simulink model "AutomotiveEMS"  (R2018a)
settings: Solver=VariableStepAuto  StartTime=0  StopTime=3.5  FixedStep=1e-6
undefined symbols (not defined in the file): alternator, buck, DiscIntNeverNeededParam, electrical_load, hybrid_control, i_f_max, iceToAltRotRatio, n_ice_f, n_ice_i, rectifier, t_brake_f, t_brake_i, T_k, T_r, T_s
libraries: fl_lib x43, nesl_utility x41, elec_lib x33, simulink x10, SimscapeCustomBlocks_lib x2, dsparch4 x2, pe_lib x1
(part 2 of 3)

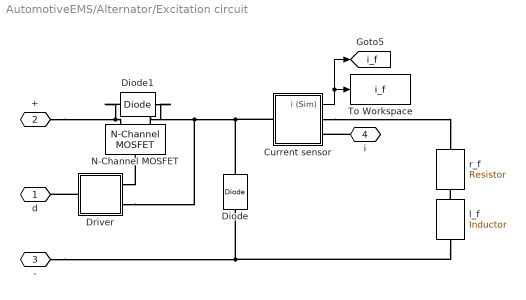
== system AutomotiveEMS/Alternator/Excitation circuit ==
  Current sensor : Subsystem
  Diode : elec_lib/Semiconductor Devices/Diode  ModelType=1  Vf=0.8 V  Ron=10e-3 Ohm  Goff=1e-8 S  Rz=0.3 Ohm  Vz=50 V  C_PWL=5 pF  prmExp=1  I12=[.0137, .545] A  V12=[.6, .7] V  I1=0.0137 A  V1=0.6 V  IS=1e-12 A  ec=1  RS=0.01 Ohm  Tmeas=25 degC  BV=inf V  C_param=1  CJ0=5 pF  VJ=1 V  Mgrad=0.5  Vvec=[.1, 10, 100] V  Cvec=[3.5, 1, .4] pF  FC=0.5  Q_param=1  Irrm=-7.15 A  iF=4 A  didt=-750 A/us  trr=115 ns  TT=50 ns  tau=100 ns  T_param=1  IS_T2=1.25e-7 A  I1_T2=0.245 A  V1_T2=0.5 V  Tmeas2=125 degC  EG_param=1  EG=1.11 eV  XTI_param=1  XTI=3  dBVdT=0 V/K  Tdevice=25 degC  i_capacitor_specify=off  i_capacitor_priority=High  i_capacitor=0 A  i_capacitor_nominal_specify=off  i_capacitor_nominal_unit=A  i_capacitor_nominal_value=1  v_capacitor_specify=off  v_capacitor_priority=None  v_capacitor=0 V  v_capacitor_nominal_specify=off  v_capacitor_nominal_unit=V  v_capacitor_nominal_value=1  Rth=[0, 10] K/W  thermal_mass_parameterization=1  thermal_mass=[0, 1] J/K  thermal_time_constant=[0, 10] s  thermal_mass_initial_temperatures=[25, 25] degC
      settings: SourceProductName=Simscape Electronics  SourceProductBaseCode=SN
  Diode1 : elec_lib/Semiconductor Devices/Diode  ModelType=1  Vf=0.8 V  Ron=10e-3 Ohm  Goff=1e-8 S  Rz=0.3 Ohm  Vz=50 V  C_PWL=5 pF  prmExp=1  I12=[.0137, .545] A  V12=[.6, .7] V  I1=0.0137 A  V1=0.6 V  IS=1e-12 A  ec=1  RS=0.01 Ohm  Tmeas=25 degC  BV=inf V  C_param=1  CJ0=5 pF  VJ=1 V  Mgrad=0.5  Vvec=[.1, 10, 100] V  Cvec=[3.5, 1, .4] pF  FC=0.5  Q_param=1  Irrm=-7.15 A  iF=4 A  didt=-750 A/us  trr=115 ns  TT=50 ns  tau=100 ns  T_param=1  IS_T2=1.25e-7 A  I1_T2=0.245 A  V1_T2=0.5 V  Tmeas2=125 degC  EG_param=1  EG=1.11 eV  XTI_param=1  XTI=3  dBVdT=0 V/K  Tdevice=25 degC  i_capacitor_specify=off  i_capacitor_priority=High  i_capacitor=0 A  i_capacitor_nominal_specify=off  i_capacitor_nominal_unit=A  i_capacitor_nominal_value=1  v_capacitor_specify=off  v_capacitor_priority=None  v_capacitor=0 V  v_capacitor_nominal_specify=off  v_capacitor_nominal_unit=V  v_capacitor_nominal_value=1  Rth=[0, 10] K/W  thermal_mass_parameterization=1  thermal_mass=[0, 1] J/K  thermal_time_constant=[0, 10] s  thermal_mass_initial_temperatures=[25, 25] degC
      settings: SourceProductName=Simscape Electronics  SourceProductBaseCode=SN
  Driver : Subsystem
  N-Channel MOSFET : elec_lib/Semiconductor Devices/N-Channel MOSFET  parameterization=1  prmDatasheet=1  prmEquCoeff=1  Beta=5 A/V^2  Rds=0.025 Ohm  Id=6 A  Vgs=alternator.rotor.s.v_gs_on V  Vth=1.7 V  lam=0 1/V  Tmeas=25 degC  RS=1e-4 Ohm  RD=0.01 Ohm  C_param=1  C_GS=270 pF  C_GD=80 pF  C_DS=0 pF  C_iss=350 pF  C_rss=80 pF  C_oss=0 pF  C_GS_vec=[ 270 300 290 280 295 255 ] pF  C_GD_vec=[ 450 400 300 190 95 55 ] pF  C_DS_vec=[ 450 410 390 230 175 115 ] pF  C_iss_vec=[ 720 700 590 470 390 310 ] pF  C_rss_vec=[ 450 400 300 190 95 55 ] pF  C_oss_vec=[ 900 810 690 420 270 170 ] pF  C_Vds_vec=[ 0.1 0.3 1 3 10 30 ] V  V_GS_for_cap_data=0 V  charge_linearity_param=1  C_OX=200 pF  V_C_OX=-0.5 V  IsDiode=0 A  Vbi=0.6 V  n=1  Cj0Diode=0 pF  TT=50e-9 s  dVth_dT=-6 mV/K  Rds_T2=0.037 Ohm  Tmeas2=125 degC  BEXDatasheet=-1.5  BEXEquCoeff=-1.5  etaisDatasheet=3  etaisEquCoeff=3  TdeviceDatasheet=25 degC  TdeviceEquCoeff=25 degC  Rth=[1, 10] K/W  thermal_mass_parameterization=1  thermal_mass=[1, 1] J/K  thermal_time_constant=[1, 10] s  thermal_mass_initial_temperatures=[ 25 25 ] degC  betaref=18 A/V^2  Vfbref=-1.1 V  gamma=3.5 V^0.50000  phib2ref=1 V  thesatref=0.4 1/V  alpha=0  Vp=5e-2 V  thesrref=0 1/V  m=8  Tref=25 degC  Cox=1500 pF  Cgso=100 pF  Cgdo=14 pF  Rsref=2e-3 Ohm  Rdref=0.17 Ohm  Rgref=8.4 Ohm  Isref=5.2e-13 A  Cj0=480 pF  Tprm=1  etabet=1.3  Stvfb=5e-4 V/K  Stphib=-8.5e-4 V/K  etasat=1.04  etasr=0.65  etar=0.95  etais=3  Tsim=25 degC  T0=[25, 25] degC
      settings: SourceProductName=Simscape Electronics  SourceProductBaseCode=SN
  To Workspace : ToWorkspace  VariableName=i_f  SaveFormat=Timeseries  SampleTime=-1
  l_f : elec_lib/Passive Devices/Inductor  l=alternator.rotor.l.value H  L_tol=20  enable_L_tol=0  tol_distribution=1  nSigma=4  r=0 Ohm  g=1e-9 1/Ohm  enable_operating_limits=0  operating_limit_action=2  max_working_current=1 A  power_rating=1 W  enable_faults=0  fault_action=1  lambdaPercent=50  k_faulted=0.9999  turnsShort=0  openCct=0  groundShort=0  groundShortG=0 1/Ohm  tau_fault=1e-3 s  enable_temporal_fault=0  t_fault=1 s  enable_behavioral_fault=0  max_permissible_voltage=100 V  n_fail_on_voltage=1  max_permissible_current=1 A  t_fail_on_current=1 s  i_L_specify=off  i_L_priority=High  i_L=0 A  i_L_nominal_specify=off  i_L_nominal_unit=A  i_L_nominal_value=1
      settings: SourceProductName=Simscape Electronics  SourceProductBaseCode=SN
  r_f : elec_lib/Passive Devices/Resistor  R=alternator.rotor.r.value Ohm  R_tol=5  enable_R_tol=0  tol_distribution=1  nSigma=4  enable_operating_limits=0  operating_limit_action=2  max_working_voltage=100 V  power_rating=1 W  enable_faults=0  fault_action=1  R_faulted=inf Ohm  enable_temporal_fault=0  t_fault=1 s  enable_behavioral_fault=0  max_permissible_current=1 A  t_fail_on_current=1 s  noise_mode=0  sample_time=1e-3 s  repeatability=1  auto_seed=2348512679  user_seed=0  Tdevice=25 degC  alpha=3.93e-3 1/K  Tmeas=25 degC  thermal_mass=100 J/K  power_derating_T1=70 degC  power_derating_T2=155 degC  operating_temperature_range_vec=[-50.0, 150.0] degC  temperature_specify=off  temperature_priority=High  temperature=298.15 K  temperature_nominal_specify=off  temperature_nominal_unit=K  temperature_nominal_value=1
  d : PMIOPort  Side=Left
  + : PMIOPort  Port=2  Side=Left
  - : PMIOPort  Port=3  Side=Left
  i : PMIOPort  Port=4  Side=Right
  tag scope: i_f=global
  wires:
  Current sensor/1(i (Sim)) -> [i_f], To Workspace/1
  connections:
  l_f/RConn1 -- Diode/LConn1 -- -/RConn1
  +/RConn1 -- Diode1/RConn1 -- N-Channel MOSFET/RConn1
  Current sensor/RConn1 -- r_f/RConn1
  Current sensor/LConn1 -- Diode/RConn1 -- Driver/RConn2 -- Diode1/LConn1 -- N-Channel MOSFET/RConn2
  l_f/LConn1 -- r_f/LConn1
  Driver/RConn1 -- N-Channel MOSFET/LConn1
  i/RConn1 -- Current sensor/RConn2
  Driver/LConn1 -- d/RConn1

== system AutomotiveEMS/Hybrid Load Matching Controller Scheme/Excitation current controller ==
  e : Inport
  on : Inport  Port=2
  Constant : Constant
  Fcn : Fcn  Expr=u > 0
  Switch : Switch  Criteria=u2 > Threshold  Threshold=0.5
  u : Outport
  wires:
  Switch/1 -> u/1
  on/1 -> Switch/2
  Constant/1 -> Switch/3
  Fcn/1 -> Switch/1
  e/1 -> Fcn/1

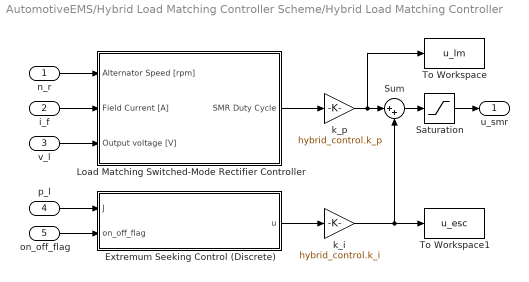
== system AutomotiveEMS/Hybrid Load Matching Controller Scheme/Hybrid Load Matching Controller ==
  n_r : Inport
  i_f : Inport  Port=2
  v_l : Inport  Port=3
  p_l : Inport  Port=4
  on_off_flag : Inport  Port=5
  Extremum Seeking Control (Discrete) : Subsystem  mask{a=0.025, f=sqrt(100*200), phi=180 - 4.2e-3/(1/sqrt(100*200))*360, K=0.25}
      mask prompts: a "Sine wave gain"; f "Sine wave frequency [Hz]"; phi "Sine wave phase [deg]"; K "Integrator gain"
      mask DialogControl ModParam Prompt: Modulation
      mask DialogControl IntegratorParam Prompt: Integrator
  Load Matching Switched-Mode Rectifier Controller : Subsystem  VariantControl=Variant  mask{p=alternator.p, u_lim_l=0.0, u_lim_u=1}
      mask prompts: p "Pole-pairs"; u_lim_l "Control signal lower limit"; u_lim_u "Control signal upper limit"
  Saturation : Saturate  UpperLimit=0.9  LowerLimit=0
  Sum : Sum  Inputs=|++
  To Workspace : ToWorkspace  VariableName=u_lm  SaveFormat=Timeseries  SampleTime=-1
  To Workspace1 : ToWorkspace  VariableName=u_esc  SaveFormat=Timeseries  SampleTime=-1
  k_i : Gain  Gain=hybrid_control.k_i
  k_p : Gain  Gain=hybrid_control.k_p
  u_smr : Outport
  wires:
  Extremum Seeking Control (Discrete)/1(u) -> k_i/1
  on_off_flag/1 -> Extremum Seeking Control (Discrete)/2(on_off_flag)
  i_f/1 -> Load Matching Switched-Mode Rectifier Controller/2(Field Current [A])
  Sum/1 -> Saturation/1
  Load Matching Switched-Mode Rectifier Controller/1(SMR Duty Cycle) -> k_p/1
  p_l/1 -> Extremum Seeking Control (Discrete)/1(J)
  v_l/1 -> Load Matching Switched-Mode Rectifier Controller/3(Output voltage [V])
  n_r/1 -> Load Matching Switched-Mode Rectifier Controller/1(Alternator Speed [rpm])
  Saturation/1 -> u_smr/1
  k_p/1 -> To Workspace/1, Sum/1
  k_i/1 -> To Workspace1/1, Sum/2

== system AutomotiveEMS/Mechanical speed/ICE Speed ==
  Ramp off : simulink/Sources/Ramp  slope=(s_f - s_i)/(t_f - t_i)  start=t_f  InitialOutput=0
  Ramp on : simulink/Sources/Ramp  slope=(s_f - s_i)/(t_f - t_i)  start=t_i  InitialOutput=s_i
  Sum : Sum  Inputs=+-
  s : Outport
  wires:
  Sum/1 -> s/1
  Ramp off/1 -> Sum/2
  Ramp on/1 -> Sum/1

== system AutomotiveEMS/Three-phase switched rectifier/Driver (S1) ==
  Controlled PWM Voltage : elec_lib/Actuators & Drivers/Drivers/Controlled PWM Voltage  F=rectifier.control.pwm.f_s Hz  TD=0 s  pulse_width_offset=0 s  pulse_min=0 s  Vmin=0 V  Vmax=5 V  Vm=5 V  pwm_or_av=1  event_type=2  sample_time=T_s s  u_min=0  u_max=1
      settings: SourceProductName=Simscape Electronics  SourceProductBaseCode=SN
  Electrical Reference : fl_lib/Electrical/Electrical Elements/Electrical Reference
  Gate Driver : elec_lib/Actuators & Drivers/Drivers/Gate Driver  vHigh=rectifier.s.v_gs_on*1.5 V  vLow=0 V  parameterization=1  rHigh=100 Ohm  rLow=10 Ohm  tRise=20 ns  tFall=20 ns  cLoad=10 nF  enable_faults=0  t_fault=1 s  fault_type=1  uHighValue=0.7  uLowValue=0.3  tHigh=50 ns  tLow=100 ns  ZonTime_specify=off  ZonTime_priority=None  ZonTime=0 s  ZoffTime_specify=off  ZoffTime_priority=None  ZoffTime=0 s  uHigh=2.0 V  uLow=0.8 V
      settings: SourceProductName=Simscape Electronics  SourceProductBaseCode=SN
  d : PMIOPort  Side=Left
  v_g : PMIOPort  Port=2  Side=Right
  v_s : PMIOPort  Port=3  Side=Right
  connections:
  Gate Driver/LConn2 -- Controlled PWM Voltage/RConn2 -- Electrical Reference/LConn1
  Controlled PWM Voltage/RConn1 -- Gate Driver/LConn1
  v_g/RConn1 -- Gate Driver/RConn1
  v_s/RConn1 -- Gate Driver/RConn2
  d/RConn1 -- Controlled PWM Voltage/LConn1

== system AutomotiveEMS/Three-phase switched rectifier/Driver (S2) ==
  Controlled PWM Voltage : elec_lib/Actuators & Drivers/Drivers/Controlled PWM Voltage  F=rectifier.control.pwm.f_s Hz  TD=0 s  pulse_width_offset=0 s  pulse_min=0 s  Vmin=0 V  Vmax=5 V  Vm=5 V  pwm_or_av=1  event_type=2  sample_time=T_s s  u_min=0  u_max=1
      settings: SourceProductName=Simscape Electronics  SourceProductBaseCode=SN
  Electrical Reference : fl_lib/Electrical/Electrical Elements/Electrical Reference
  Gate Driver : elec_lib/Actuators & Drivers/Drivers/Gate Driver  vHigh=rectifier.s.v_gs_on*1.5 V  vLow=0 V  parameterization=1  rHigh=100 Ohm  rLow=10 Ohm  tRise=20 ns  tFall=20 ns  cLoad=10 nF  enable_faults=0  t_fault=1 s  fault_type=1  uHighValue=0.7  uLowValue=0.3  tHigh=50 ns  tLow=100 ns  ZonTime_specify=off  ZonTime_priority=None  ZonTime=0 s  ZoffTime_specify=off  ZoffTime_priority=None  ZoffTime=0 s  uHigh=2.0 V  uLow=0.8 V
      settings: SourceProductName=Simscape Electronics  SourceProductBaseCode=SN
  d : PMIOPort  Side=Left
  v_g : PMIOPort  Port=2  Side=Right
  v_s : PMIOPort  Port=3  Side=Right
  connections:
  Gate Driver/LConn2 -- Controlled PWM Voltage/RConn2 -- Electrical Reference/LConn1
  Controlled PWM Voltage/RConn1 -- Gate Driver/LConn1
  v_g/RConn1 -- Gate Driver/RConn1
  v_s/RConn1 -- Gate Driver/RConn2
  d/RConn1 -- Controlled PWM Voltage/LConn1

== system AutomotiveEMS/Three-phase switched rectifier/Driver (S3) ==
  Controlled PWM Voltage : elec_lib/Actuators & Drivers/Drivers/Controlled PWM Voltage  F=rectifier.control.pwm.f_s Hz  TD=0 s  pulse_width_offset=0 s  pulse_min=0 s  Vmin=0 V  Vmax=5 V  Vm=5 V  pwm_or_av=1  event_type=2  sample_time=T_s s  u_min=0  u_max=1
      settings: SourceProductName=Simscape Electronics  SourceProductBaseCode=SN
  Electrical Reference : fl_lib/Electrical/Electrical Elements/Electrical Reference
  Gate Driver : elec_lib/Actuators & Drivers/Drivers/Gate Driver  vHigh=rectifier.s.v_gs_on*1.5 V  vLow=0 V  parameterization=1  rHigh=100 Ohm  rLow=10 Ohm  tRise=20 ns  tFall=20 ns  cLoad=10 nF  enable_faults=0  t_fault=1 s  fault_type=1  uHighValue=0.7  uLowValue=0.3  tHigh=50 ns  tLow=100 ns  ZonTime_specify=off  ZonTime_priority=None  ZonTime=0 s  ZoffTime_specify=off  ZoffTime_priority=None  ZoffTime=0 s  uHigh=2.0 V  uLow=0.8 V
      settings: SourceProductName=Simscape Electronics  SourceProductBaseCode=SN
  d : PMIOPort  Side=Left
  v_g : PMIOPort  Port=2  Side=Right
  v_s : PMIOPort  Port=3  Side=Right
  connections:
  Gate Driver/LConn2 -- Controlled PWM Voltage/RConn2 -- Electrical Reference/LConn1
  Controlled PWM Voltage/RConn1 -- Gate Driver/LConn1
  v_g/RConn1 -- Gate Driver/RConn1
  v_s/RConn1 -- Gate Driver/RConn2
  d/RConn1 -- Controlled PWM Voltage/LConn1

== system AutomotiveEMS/i_bus sensor/Current Sensor ==
  Ideal current sensor : Subsystem
  Noise addition : Subsystem  mask{T_s=T_s, seed=seed, noise=noise}
      mask prompts: T_s "Sample time [s]"; noise "Noise percentage"
  + : PMIOPort  Side=Left
  - : PMIOPort  Port=2  Side=Right
  m* : Outport
  m : Outport  Port=2
  wires:
  Ideal current sensor/1(i) -> m*/1, Noise addition/1(u)
  Noise addition/1(u + n) -> m/1
  connections:
  Ideal current sensor/RConn1 -- -/RConn1
  Ideal current sensor/LConn1 -- +/RConn1

== system AutomotiveEMS/i_l sensor/Current Sensor ==
  Ideal current sensor : Subsystem
  Noise addition : Subsystem  mask{T_s=T_s, seed=seed, noise=noise}
      mask prompts: T_s "Sample time [s]"; noise "Noise percentage"
  + : PMIOPort  Side=Left
  - : PMIOPort  Port=2  Side=Right
  m* : Outport
  m : Outport  Port=2
  wires:
  Ideal current sensor/1(i) -> m*/1, Noise addition/1(u)
  Noise addition/1(u + n) -> m/1
  connections:
  Ideal current sensor/RConn1 -- -/RConn1
  Ideal current sensor/LConn1 -- +/RConn1

== system AutomotiveEMS/i_uc sensor/Current Sensor ==
  Ideal current sensor : Subsystem
  Noise addition : Subsystem  mask{T_s=T_s, seed=seed, noise=noise}
      mask prompts: T_s "Sample time [s]"; noise "Noise percentage"
  + : PMIOPort  Side=Left
  - : PMIOPort  Port=2  Side=Right
  m* : Outport
  m : Outport  Port=2
  wires:
  Ideal current sensor/1(i) -> m*/1, Noise addition/1(u)
  Noise addition/1(u + n) -> m/1
  connections:
  Ideal current sensor/RConn1 -- -/RConn1
  Ideal current sensor/LConn1 -- +/RConn1

== system AutomotiveEMS/n_r sensor/Noise addition ==
  u : Inport
  Band-Limited White Noise : simulink/Sources/Band-Limited White Noise  Cov=[0.1]  Ts=T_s  seed=[seed]
  Gain : Gain  Gain=1/100
  Gain3 : Gain  Gain=noise
  Product2 : Product
  Sum1 : Sum  Inputs=|++
  Zero-Order Hold : ZeroOrderHold  SampleTime=T_s
  u + n : Outport
  wires:
  Gain3/1 -> Product2/1
  Product2/1 -> Sum1/1
  Gain/1 -> Product2/2
  u/1 -> Sum1/2, Gain3/1
  Band-Limited White Noise/1 -> Gain/1
  Sum1/1 -> Zero-Order Hold/1
  Zero-Order Hold/1 -> u + n/1

== system AutomotiveEMS/v_bus sensor/Voltage Sensor ==
  Ideal voltage sensor : Subsystem
  Noise addition : Subsystem  mask{T_s=T_s, seed=seed, noise=noise}
      mask prompts: T_s "Sample time [s]"; noise "Noise percentage"
  + : PMIOPort  Side=Left
  - : PMIOPort  Port=2  Side=Left
  m* : Outport
  m : Outport  Port=2
  wires:
  Ideal voltage sensor/1(v) -> m*/1, Noise addition/1(u)
  Noise addition/1(u + n) -> m/1
  connections:
  Ideal voltage sensor/LConn1 -- +/RConn1
  Ideal voltage sensor/RConn1 -- -/RConn1

== system AutomotiveEMS/v_l sensor/Voltage Sensor ==
  Ideal voltage sensor : Subsystem
  Noise addition : Subsystem  mask{T_s=T_s, seed=seed, noise=noise}
      mask prompts: T_s "Sample time [s]"; noise "Noise percentage"
  + : PMIOPort  Side=Left
  - : PMIOPort  Port=2  Side=Left
  m* : Outport
  m : Outport  Port=2
  wires:
  Ideal voltage sensor/1(v) -> m*/1, Noise addition/1(u)
  Noise addition/1(u + n) -> m/1
  connections:
  Ideal voltage sensor/LConn1 -- +/RConn1
  Ideal voltage sensor/RConn1 -- -/RConn1

== system AutomotiveEMS/v_uc sensor/Voltage Sensor ==
  Ideal voltage sensor : Subsystem
  Noise addition : Subsystem  mask{T_s=T_s, seed=seed, noise=noise}
      mask prompts: T_s "Sample time [s]"; noise "Noise percentage"
  + : PMIOPort  Side=Left
  - : PMIOPort  Port=2  Side=Left
  m* : Outport
  m : Outport  Port=2
  wires:
  Ideal voltage sensor/1(v) -> m*/1, Noise addition/1(u)
  Noise addition/1(u + n) -> m/1
  connections:
  Ideal voltage sensor/LConn1 -- +/RConn1
  Ideal voltage sensor/RConn1 -- -/RConn1

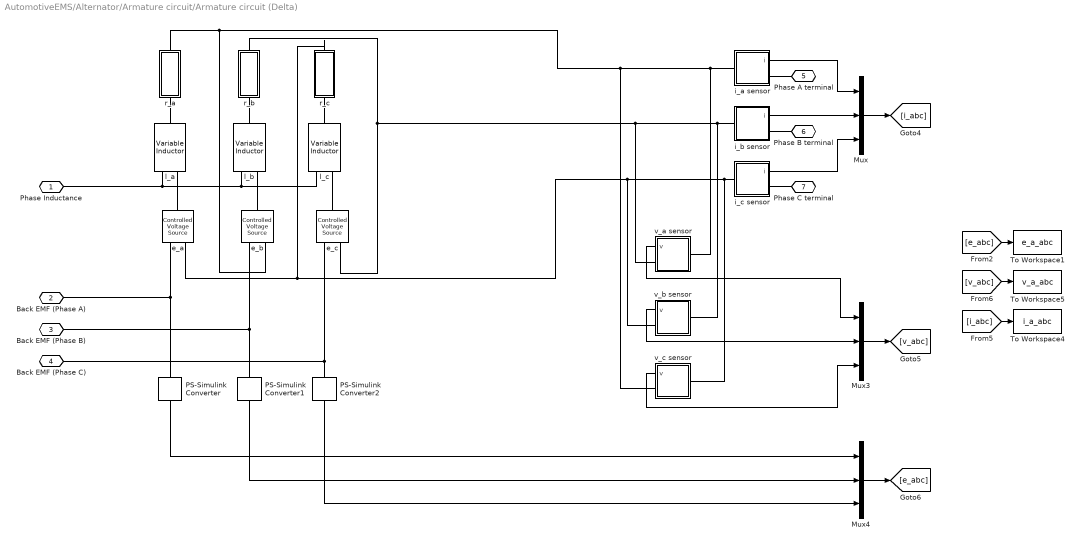
== system AutomotiveEMS/Alternator/Armature circuit/Armature circuit (Delta) ==
  Mux : Mux  Inputs=3
  Mux3 : Mux  Inputs=3
  Mux4 : Mux  Inputs=3
  PS-Simulink Converter : nesl_utility/PS-Simulink Converter  PhysicalDomain=network_engine_domain  SubClassName=ps_output  LeftPortType=input  RightPortType=output  PseudoPeriodic=off  Frequencies=[]  Unit=1  AffineConversion=off
  PS-Simulink Converter1 : nesl_utility/PS-Simulink Converter  PhysicalDomain=network_engine_domain  SubClassName=ps_output  LeftPortType=input  RightPortType=output  PseudoPeriodic=off  Frequencies=[]  Unit=1  AffineConversion=off
  PS-Simulink Converter2 : nesl_utility/PS-Simulink Converter  PhysicalDomain=network_engine_domain  SubClassName=ps_output  LeftPortType=input  RightPortType=output  PseudoPeriodic=off  Frequencies=[]  Unit=1  AffineConversion=off
  To Workspace1 : ToWorkspace  VariableName=e_a_abc  SaveFormat=Timeseries  SampleTime=-1
  To Workspace4 : ToWorkspace  VariableName=i_a_abc  SaveFormat=Timeseries  SampleTime=-1
  To Workspace5 : ToWorkspace  VariableName=v_a_abc  SaveFormat=Timeseries  SampleTime=-1
  e_a : fl_lib/Electrical/Electrical Sources/Controlled Voltage Source
  e_b : fl_lib/Electrical/Electrical Sources/Controlled Voltage Source
  e_c : fl_lib/Electrical/Electrical Sources/Controlled Voltage Source
  i_a sensor : Subsystem
  i_b sensor : Subsystem
  i_c sensor : Subsystem
  l_a : elec_lib/Passive Devices/Variable Inductor  prm=1  Lmin=1e-6 H  g=1e-9 1/Ohm  i0=0 A  phi0=0 Wb
      settings: SourceProductName=Simscape Electronics  SourceProductBaseCode=SN
  l_b : elec_lib/Passive Devices/Variable Inductor  prm=1  Lmin=1e-6 H  g=1e-9 1/Ohm  i0=0 A  phi0=0 Wb
      settings: SourceProductName=Simscape Electronics  SourceProductBaseCode=SN
  l_c : elec_lib/Passive Devices/Variable Inductor  prm=1  Lmin=1e-6 H  g=1e-9 1/Ohm  i0=0 A  phi0=0 Wb
      settings: SourceProductName=Simscape Electronics  SourceProductBaseCode=SN
  r_a : Subsystem  mask{r_ref=alternator.stator.r.value, T_ref=alternator.stator.r.T_ref, T=alternator.stator.r.T, alpha=alternator.stator.r.alpha}
      mask prompts: r_ref "Nominal resistance [Ohm]"; T_ref "Reference temperature [oC]"; T "Resistor temperature [oC]"; alpha "Temperature Coefficient [1/oC]"
  r_b : Subsystem  mask{r_ref=alternator.stator.r.value, T_ref=alternator.stator.r.T_ref, T=alternator.stator.r.T, alpha=alternator.stator.r.alpha}
      mask prompts: r_ref "Nominal resistance [Ohm]"; T_ref "Reference temperature [oC]"; T "Resistor temperature [oC]"; alpha "Temperature Coefficient [1/oC]"
  r_c : Subsystem  mask{r_ref=alternator.stator.r.value, T_ref=alternator.stator.r.T_ref, T=alternator.stator.r.T, alpha=alternator.stator.r.alpha}
      mask prompts: r_ref "Nominal resistance [Ohm]"; T_ref "Reference temperature [oC]"; T "Resistor temperature [oC]"; alpha "Temperature Coefficient [1/oC]"
  v_a sensor : Subsystem
  v_b sensor : Subsystem
  v_c sensor : Subsystem
  Phase Inductance : PMIOPort  Side=Left
  Back EMF (Phase A) : PMIOPort  Port=2  Side=Left
  Back EMF (Phase B) : PMIOPort  Port=3  Side=Left
  Back EMF (Phase C) : PMIOPort  Port=4  Side=Left
  Phase A terminal : PMIOPort  Port=5  Side=Right
  Phase B terminal : PMIOPort  Port=6  Side=Right
  Phase C terminal : PMIOPort  Port=7  Side=Right
  wires:
  [i_abc] -> To Workspace4/1
  [v_abc] -> To Workspace5/1
  [e_abc] -> To Workspace1/1
  i_c sensor/1(i) -> Mux/3
  Mux4/1 -> [e_abc]
  v_b sensor/1(v) -> Mux3/2
  v_c sensor/1(v) -> Mux3/3
  PS-Simulink Converter2/1 -> Mux4/3
  PS-Simulink Converter1/1 -> Mux4/2
  v_a sensor/1(v) -> Mux3/1
  Mux/1 -> [i_abc]
  i_b sensor/1(i) -> Mux/2
  PS-Simulink Converter/1 -> Mux4/1
  i_a sensor/1(i) -> Mux/1
  Mux3/1 -> [v_abc]
  connections:
  l_c/LConn1 -- l_b/LConn1 -- l_a/LConn1 -- Phase Inductance/RConn1
  r_b/RConn1 -- v_a sensor/RConn1 -- i_b sensor/LConn1 -- v_b sensor/LConn1 -- e_c/RConn2
  v_b sensor/RConn1 -- e_a/RConn2 -- r_c/RConn1 -- v_c sensor/LConn1 -- i_c sensor/LConn1
  PS-Simulink Converter1/LConn1 -- Back EMF (Phase B)/RConn1 -- e_b/RConn1
  r_a/RConn1 -- e_b/RConn2 -- v_a sensor/LConn1 -- i_a sensor/LConn1 -- v_c sensor/RConn1
  PS-Simulink Converter2/LConn1 -- Back EMF (Phase C)/RConn1 -- e_c/RConn1
  PS-Simulink Converter/LConn1 -- Back EMF (Phase A)/RConn1 -- e_a/RConn1
  r_c/LConn1 -- l_c/RConn1
  i_a sensor/RConn1 -- Phase A terminal/RConn1
  i_c sensor/RConn1 -- Phase C terminal/RConn1
  e_a/LConn1 -- l_a/LConn2
  r_b/LConn1 -- l_b/RConn1
  r_a/LConn1 -- l_a/RConn1
  e_b/LConn1 -- l_b/LConn2
  e_c/LConn1 -- l_c/LConn2
  i_b sensor/RConn1 -- Phase B terminal/RConn1

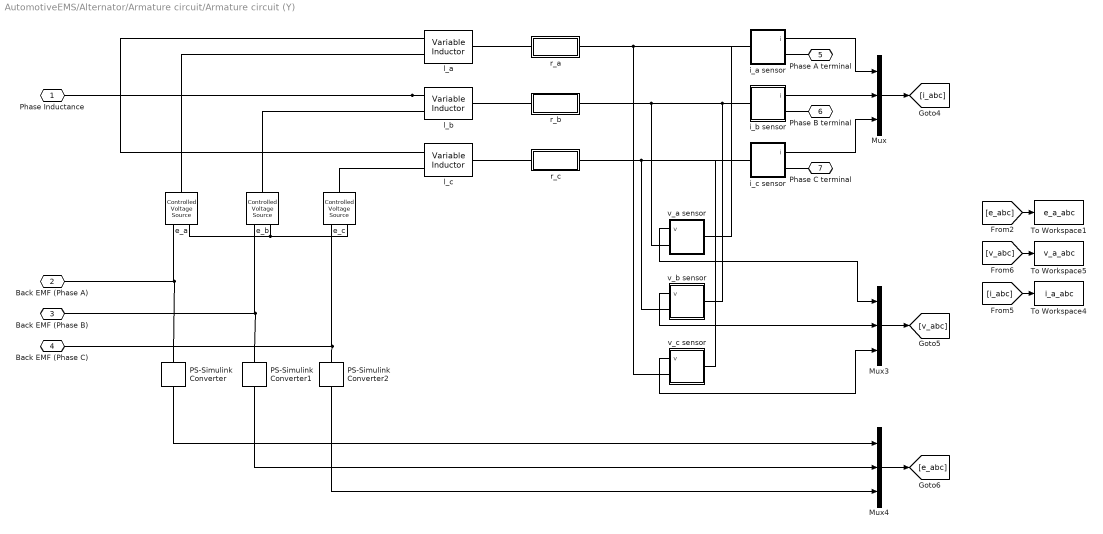
== system AutomotiveEMS/Alternator/Armature circuit/Armature circuit (Y) ==
  Mux : Mux  Inputs=3
  Mux3 : Mux  Inputs=3
  Mux4 : Mux  Inputs=3
  PS-Simulink Converter : nesl_utility/PS-Simulink Converter  PhysicalDomain=network_engine_domain  SubClassName=ps_output  LeftPortType=input  RightPortType=output  PseudoPeriodic=off  Frequencies=[]  Unit=1  AffineConversion=off
  PS-Simulink Converter1 : nesl_utility/PS-Simulink Converter  PhysicalDomain=network_engine_domain  SubClassName=ps_output  LeftPortType=input  RightPortType=output  PseudoPeriodic=off  Frequencies=[]  Unit=1  AffineConversion=off
  PS-Simulink Converter2 : nesl_utility/PS-Simulink Converter  PhysicalDomain=network_engine_domain  SubClassName=ps_output  LeftPortType=input  RightPortType=output  PseudoPeriodic=off  Frequencies=[]  Unit=1  AffineConversion=off
  To Workspace1 : ToWorkspace  VariableName=e_a_abc  SaveFormat=Timeseries  SampleTime=-1
  To Workspace4 : ToWorkspace  VariableName=i_a_abc  SaveFormat=Timeseries  SampleTime=-1
  To Workspace5 : ToWorkspace  VariableName=v_a_abc  SaveFormat=Timeseries  SampleTime=-1
  e_a : fl_lib/Electrical/Electrical Sources/Controlled Voltage Source
  e_b : fl_lib/Electrical/Electrical Sources/Controlled Voltage Source
  e_c : fl_lib/Electrical/Electrical Sources/Controlled Voltage Source
  i_a sensor : Subsystem
  i_b sensor : Subsystem
  i_c sensor : Subsystem
  l_a : elec_lib/Passive Devices/Variable Inductor  prm=1  Lmin=1e-6 H  g=1e-9 1/Ohm  i0=0 A  phi0=0 Wb
      settings: SourceProductName=Simscape Electronics  SourceProductBaseCode=SN
  l_b : elec_lib/Passive Devices/Variable Inductor  prm=1  Lmin=1e-6 H  g=1e-9 1/Ohm  i0=0 A  phi0=0 Wb
      settings: SourceProductName=Simscape Electronics  SourceProductBaseCode=SN
  l_c : elec_lib/Passive Devices/Variable Inductor  prm=1  Lmin=1e-6 H  g=1e-9 1/Ohm  i0=0 A  phi0=0 Wb
      settings: SourceProductName=Simscape Electronics  SourceProductBaseCode=SN
  r_a : Subsystem  mask{r_ref=alternator.stator.r.value, T_ref=alternator.stator.r.T_ref, T=alternator.stator.r.T, alpha=alternator.stator.r.alpha}
      mask prompts: r_ref "Nominal resistance [Ohm]"; T_ref "Reference temperature [oC]"; T "Resistor temperature [oC]"; alpha "Temperature Coefficient [1/oC]"
  r_b : Subsystem  mask{r_ref=alternator.stator.r.value, T_ref=alternator.stator.r.T_ref, T=alternator.stator.r.T, alpha=alternator.stator.r.alpha}
      mask prompts: r_ref "Nominal resistance [Ohm]"; T_ref "Reference temperature [oC]"; T "Resistor temperature [oC]"; alpha "Temperature Coefficient [1/oC]"
  r_c : Subsystem  mask{r_ref=alternator.stator.r.value, T_ref=alternator.stator.r.T_ref, T=alternator.stator.r.T, alpha=alternator.stator.r.alpha}
      mask prompts: r_ref "Nominal resistance [Ohm]"; T_ref "Reference temperature [oC]"; T "Resistor temperature [oC]"; alpha "Temperature Coefficient [1/oC]"
  v_a sensor : Subsystem
  v_b sensor : Subsystem
  v_c sensor : Subsystem
  Phase Inductance : PMIOPort  Side=Left
  Back EMF (Phase A) : PMIOPort  Port=2  Side=Left
  Back EMF (Phase B) : PMIOPort  Port=3  Side=Left
  Back EMF (Phase C) : PMIOPort  Port=4  Side=Left
  Phase A terminal : PMIOPort  Port=5  Side=Right
  Phase B terminal : PMIOPort  Port=6  Side=Right
  Phase C terminal : PMIOPort  Port=7  Side=Right
  wires:
  [i_abc] -> To Workspace4/1
  [v_abc] -> To Workspace5/1
  [e_abc] -> To Workspace1/1
  v_c sensor/1(v) -> Mux3/3
  Mux4/1 -> [e_abc]
  PS-Simulink Converter/1 -> Mux4/1
  PS-Simulink Converter2/1 -> Mux4/3
  PS-Simulink Converter1/1 -> Mux4/2
  v_a sensor/1(v) -> Mux3/1
  v_b sensor/1(v) -> Mux3/2
  i_b sensor/1(i) -> Mux/2
  Mux/1 -> [i_abc]
  i_a sensor/1(i) -> Mux/1
  Mux3/1 -> [v_abc]
  i_c sensor/1(i) -> Mux/3
  connections:
  PS-Simulink Converter/LConn1 -- e_a/RConn1 -- Back EMF (Phase A)/RConn1
  l_b/LConn1 -- l_a/LConn1 -- Phase Inductance/RConn1 -- l_c/LConn1
  r_b/RConn1 -- v_a sensor/RConn1 -- v_b sensor/LConn1 -- i_b sensor/LConn1
  r_c/RConn1 -- i_c sensor/LConn1 -- v_c sensor/LConn1 -- v_b sensor/RConn1
  PS-Simulink Converter2/LConn1 -- e_c/RConn1 -- Back EMF (Phase C)/RConn1
  r_a/RConn1 -- i_a sensor/LConn1 -- v_a sensor/LConn1 -- v_c sensor/RConn1
  PS-Simulink Converter1/LConn1 -- e_b/RConn1 -- Back EMF (Phase B)/RConn1
  e_b/RConn2 -- e_a/RConn2 -- e_c/RConn2
  i_b sensor/RConn1 -- Phase B terminal/RConn1
  i_a sensor/RConn1 -- Phase A terminal/RConn1
  e_c/LConn1 -- l_c/LConn2
  i_c sensor/RConn1 -- Phase C terminal/RConn1
  e_a/LConn1 -- l_a/LConn2
  r_c/LConn1 -- l_c/RConn1
  e_b/LConn1 -- l_b/LConn2
  r_b/LConn1 -- l_b/RConn1
  r_a/LConn1 -- l_a/RConn1

== system AutomotiveEMS/Alternator/Excitation circuit/Current sensor ==
  Current Sensor1 : fl_lib/Electrical/Electrical Sensors/Current Sensor
  PS-Simulink Converter1 : nesl_utility/PS-Simulink Converter  PhysicalDomain=network_engine_domain  SubClassName=ps_output  LeftPortType=input  RightPortType=output  PseudoPeriodic=off  Frequencies=[]  Unit=1  AffineConversion=off
  Sample delay : TransferFcn  Denominator=[T_s 1]
  + : PMIOPort  Side=Left
  - : PMIOPort  Port=2  Side=Right
  i (PS) : PMIOPort  Port=3  Side=Right
  i (Sim) : Outport
  wires:
  Sample delay/1 -> i (Sim)/1
  PS-Simulink Converter1/1 -> Sample delay/1
  connections:
  Current Sensor1/RConn2 -- -/RConn1
  Current Sensor1/LConn1 -- +/RConn1
  PS-Simulink Converter1/LConn1 -- i (PS)/RConn1 -- Current Sensor1/RConn1

== system AutomotiveEMS/Alternator/Excitation circuit/Driver ==
  Controlled PWM Voltage : elec_lib/Actuators & Drivers/Drivers/Controlled PWM Voltage  F=alternator.rotor.control.pwm.f_s Hz  TD=0 s  pulse_width_offset=0 s  pulse_min=0 s  Vmin=0 V  Vmax=5 V  Vm=5 V  pwm_or_av=1  event_type=2  sample_time=T_s s  u_min=0  u_max=1
      settings: SourceProductName=Simscape Electronics  SourceProductBaseCode=SN  LogSimulationData=on
  Electrical Reference : fl_lib/Electrical/Electrical Elements/Electrical Reference
  Gate Driver : elec_lib/Actuators & Drivers/Drivers/Gate Driver  vHigh=rectifier.s.v_gs_on*1.5 V  vLow=0 V  parameterization=1  rHigh=100 Ohm  rLow=10 Ohm  tRise=20 ns  tFall=20 ns  cLoad=10 nF  enable_faults=0  t_fault=1 s  fault_type=1  uHighValue=0.7  uLowValue=0.3  tHigh=50 ns  tLow=100 ns  ZonTime_specify=off  ZonTime_priority=None  ZonTime=0 s  ZoffTime_specify=off  ZoffTime_priority=None  ZoffTime=0 s  uHigh=2.0 V  uLow=0.8 V
      settings: SourceProductName=Simscape Electronics  SourceProductBaseCode=SN  LogSimulationData=on
  d : PMIOPort  Side=Left
  v_g : PMIOPort  Port=2  Side=Right
  v_s : PMIOPort  Port=3  Side=Right
  connections:
  Gate Driver/LConn2 -- Electrical Reference/LConn1 -- Controlled PWM Voltage/RConn2
  Controlled PWM Voltage/RConn1 -- Gate Driver/LConn1
  v_g/RConn1 -- Gate Driver/RConn1
  v_s/RConn1 -- Gate Driver/RConn2
  d/RConn1 -- Controlled PWM Voltage/LConn1

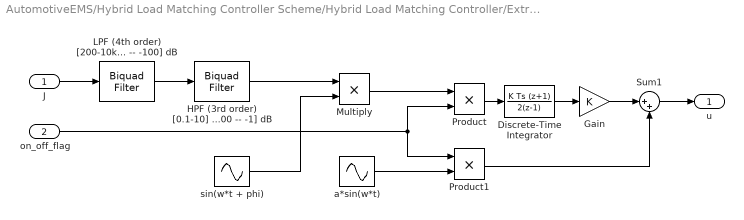
== system AutomotiveEMS/Hybrid Load Matching Controller Scheme/Hybrid Load Matching Controller/Extremum Seeking Control (Discrete) ==
  J : Inport
  on_off_flag : Inport  Port=2
  Discrete-Time Integrator : DiscreteIntegrator  IntegratorMethod=Integration: Trapezoidal  SampleTime=T_k  ICPrevOutput=DiscIntNeverNeededParam  ICPrevScaledInput=DiscIntNeverNeededParam
  Gain : Gain  Gain=K
  "HPF (3rd order) [0.1-10] Hz [-100 -- -1] dB" : dsparch4/Biquad Filter  Tag=BlockMethodSubSystem  FilterSource=Specify via dialog  CoeffSource=Specify via dialog  FilterObject=BQF  IIRFiltStruct=Direct form II  BiQuadCoeffs=[1 -2 1 1 -1.999708317857956 0.999708402899225801;1.99999999999999978 -1.99999999999999978 0 1 -0.999708402893026538 0]  ScaleValues=[8.50412698039093584e-08;1;5877783.84072393924]  IC=0  ICnum=0  ICden=0  a0Flag=Warning  optimizeScaleValues=off  ScaleValueMode=Specify via input port (g)  InputProcessing=Columns as channels (frame based)  roundingMode=Floor  overflowMode=off  scaleValueFracLength=14  denProdOutputFracLength=30  denAccumFracLength=30  secondMemoryFracLength=15
      settings: SourceProductName=DSP System Toolbox
  "LPF (4th order) [200-10k] Hz [-1 -- -100] dB" : dsparch4/Biquad Filter  Tag=BlockMethodSubSystem  FilterSource=Specify via dialog  CoeffSource=Specify via dialog  FilterObject=BQF  IIRFiltStruct=Direct form II  BiQuadCoeffs=[0.000456668121238872592 0.000913336242477745183 0.000456668121238872592 1 -1.97110934364515256 0.972425894996062246;0.250003439744055866 0.500006879488111733 0.250003439744055866 1 -1.93341199247083351 0.934703364853983421]  ScaleValues=[0.000930727690625064198;1;1]  IC=0  ICnum=0  ICden=0  a0Flag=Warning  optimizeScaleValues=off  ScaleValueMode=Specify via input port (g)  InputProcessing=Columns as channels (frame based)  roundingMode=Floor  overflowMode=off  scaleValueFracLength=14  denProdOutputFracLength=30  denAccumFracLength=30  secondMemoryFracLength=15
      settings: SourceProductName=DSP System Toolbox
  Multiply : Product
  Product : Product
  Product1 : Product
  Sum1 : Sum  Inputs=|++
  a*sin(w*t) : Sin  Amplitude=a  Frequency=2*pi*f  SampleTime=T_k
  sin(w*t + phi) : Sin  Frequency=2*pi*f  Phase=pi*phi/180  SampleTime=T_k
  u : Outport
  wires:
  Discrete-Time Integrator/1 -> Gain/1
  Gain/1 -> Sum1/1
  Sum1/1 -> u/1
  Multiply/1 -> Product/1
  on_off_flag/1 -> Product1/1, Product/2
  a*sin(w*t)/1 -> Product1/2
  sin(w*t + phi)/1 -> Multiply/2
  Product/1 -> Discrete-Time Integrator/1
  Product1/1 -> Sum1/2
  "HPF (3rd order) [0.1-10] Hz [-100 -- -1] dB"/1 -> Multiply/1
  J/1 -> "LPF (4th order) [200-10k] Hz [-1 -- -100] dB"/1
  "LPF (4th order) [200-10k] Hz [-1 -- -100] dB"/1 -> "HPF (3rd order) [0.1-10] Hz [-100 -- -1] dB"/1

== system AutomotiveEMS/Hybrid Load Matching Controller Scheme/Hybrid Load Matching Controller/Load Matching Switched-Mode Rectifier Controller ==
  Alternator Speed [rpm] : Inport
  Field Current [A] : Inport  Port=2
  Output voltage [V] : Inport  Port=3
  Lower saturation limit : Constant  Value=u_lim_l
  MATLAB Function : MATLAB Function  TreatAsAtomicUnit=on
  Pole-pairs : Constant  Value=p
  Upper saturation limit : Constant  Value=u_lim_u
  SMR Duty Cycle : Outport
  wires:
  Field Current [A]/1 -> MATLAB Function/2(i_f)
  MATLAB Function/1(u_smr) -> SMR Duty Cycle/1
  Alternator Speed [rpm]/1 -> MATLAB Function/1(n_r)
  Pole-pairs/1 -> MATLAB Function/3(p)
  Upper saturation limit/1 -> MATLAB Function/6(u_lim_u)
  Output voltage [V]/1 -> MATLAB Function/4(v_o)
  Lower saturation limit/1 -> MATLAB Function/5(u_lim_l)

== system AutomotiveEMS/i_bus sensor/Current Sensor/Ideal current sensor ==
  Current Sensor : fl_lib/Electrical/Electrical Sensors/Current Sensor
  PS-Simulink Converter : nesl_utility/PS-Simulink Converter  PhysicalDomain=network_engine_domain  SubClassName=ps_output  LeftPortType=input  RightPortType=output  PseudoPeriodic=off  Frequencies=[]  Unit=1  AffineConversion=off
  + : PMIOPort  Side=Left
  - : PMIOPort  Port=2  Side=Right
  i : Outport
  wires:
  PS-Simulink Converter/1 -> i/1
  connections:
  Current Sensor/RConn2 -- -/RConn1
  Current Sensor/LConn1 -- +/RConn1
  PS-Simulink Converter/LConn1 -- Current Sensor/RConn1

== system AutomotiveEMS/i_bus sensor/Current Sensor/Noise addition ==
  u : Inport
  Band-Limited White Noise : simulink/Sources/Band-Limited White Noise  Cov=[0.1]  Ts=T_s  seed=[seed]
  Gain : Gain  Gain=1/100
  Gain3 : Gain  Gain=noise
  Product2 : Product
  Sum1 : Sum  Inputs=|++
  Zero-Order Hold : ZeroOrderHold  SampleTime=T_s
  u + n : Outport
  wires:
  Gain3/1 -> Product2/1
  Product2/1 -> Sum1/1
  Gain/1 -> Product2/2
  u/1 -> Sum1/2, Gain3/1
  Band-Limited White Noise/1 -> Gain/1
  Sum1/1 -> Zero-Order Hold/1
  Zero-Order Hold/1 -> u + n/1

== system AutomotiveEMS/i_l sensor/Current Sensor/Ideal current sensor ==
  Current Sensor : fl_lib/Electrical/Electrical Sensors/Current Sensor
  PS-Simulink Converter : nesl_utility/PS-Simulink Converter  PhysicalDomain=network_engine_domain  SubClassName=ps_output  LeftPortType=input  RightPortType=output  PseudoPeriodic=off  Frequencies=[]  Unit=1  AffineConversion=off
  + : PMIOPort  Side=Left
  - : PMIOPort  Port=2  Side=Right
  i : Outport
  wires:
  PS-Simulink Converter/1 -> i/1
  connections:
  Current Sensor/RConn2 -- -/RConn1
  Current Sensor/LConn1 -- +/RConn1
  PS-Simulink Converter/LConn1 -- Current Sensor/RConn1

== system AutomotiveEMS/i_l sensor/Current Sensor/Noise addition ==
  u : Inport
  Band-Limited White Noise : simulink/Sources/Band-Limited White Noise  Cov=[0.1]  Ts=T_s  seed=[seed]
  Gain : Gain  Gain=1/100
  Gain3 : Gain  Gain=noise
  Product2 : Product
  Sum1 : Sum  Inputs=|++
  Zero-Order Hold : ZeroOrderHold  SampleTime=T_s
  u + n : Outport
  wires:
  Gain3/1 -> Product2/1
  Product2/1 -> Sum1/1
  Gain/1 -> Product2/2
  u/1 -> Sum1/2, Gain3/1
  Band-Limited White Noise/1 -> Gain/1
  Sum1/1 -> Zero-Order Hold/1
  Zero-Order Hold/1 -> u + n/1

== system AutomotiveEMS/i_uc sensor/Current Sensor/Ideal current sensor ==
  Current Sensor : fl_lib/Electrical/Electrical Sensors/Current Sensor
  PS-Simulink Converter : nesl_utility/PS-Simulink Converter  PhysicalDomain=network_engine_domain  SubClassName=ps_output  LeftPortType=input  RightPortType=output  PseudoPeriodic=off  Frequencies=[]  Unit=1  AffineConversion=off
  + : PMIOPort  Side=Left
  - : PMIOPort  Port=2  Side=Right
  i : Outport
  wires:
  PS-Simulink Converter/1 -> i/1
  connections:
  Current Sensor/RConn2 -- -/RConn1
  Current Sensor/LConn1 -- +/RConn1
  PS-Simulink Converter/LConn1 -- Current Sensor/RConn1

== system AutomotiveEMS/i_uc sensor/Current Sensor/Noise addition ==
  u : Inport
  Band-Limited White Noise : simulink/Sources/Band-Limited White Noise  Cov=[0.1]  Ts=T_s  seed=[seed]
  Gain : Gain  Gain=1/100
  Gain3 : Gain  Gain=noise
  Product2 : Product
  Sum1 : Sum  Inputs=|++
  Zero-Order Hold : ZeroOrderHold  SampleTime=T_s
  u + n : Outport
  wires:
  Gain3/1 -> Product2/1
  Product2/1 -> Sum1/1
  Gain/1 -> Product2/2
  u/1 -> Sum1/2, Gain3/1
  Band-Limited White Noise/1 -> Gain/1
  Sum1/1 -> Zero-Order Hold/1
  Zero-Order Hold/1 -> u + n/1

== system AutomotiveEMS/v_bus sensor/Voltage Sensor/Ideal voltage sensor ==
  PS-Simulink Converter : nesl_utility/PS-Simulink Converter  PhysicalDomain=network_engine_domain  SubClassName=ps_output  LeftPortType=input  RightPortType=output  PseudoPeriodic=off  Frequencies=[]  Unit=1  AffineConversion=off
  Voltage Sensor : fl_lib/Electrical/Electrical Sensors/Voltage Sensor
  + : PMIOPort  Side=Left
  - : PMIOPort  Port=2  Side=Right
  v : Outport
  wires:
  PS-Simulink Converter/1 -> v/1
  connections:
  Voltage Sensor/LConn1 -- +/RConn1
  -/RConn1 -- Voltage Sensor/RConn2
  Voltage Sensor/RConn1 -- PS-Simulink Converter/LConn1

== system AutomotiveEMS/v_bus sensor/Voltage Sensor/Noise addition ==
  u : Inport
  Band-Limited White Noise : simulink/Sources/Band-Limited White Noise  Cov=[0.1]  Ts=T_s  seed=[seed]
  Gain : Gain  Gain=1/100
  Gain3 : Gain  Gain=noise
  Product2 : Product
  Sum1 : Sum  Inputs=|++
  Zero-Order Hold : ZeroOrderHold  SampleTime=T_s
  u + n : Outport
  wires:
  Gain3/1 -> Product2/1
  Product2/1 -> Sum1/1
  Gain/1 -> Product2/2
  u/1 -> Sum1/2, Gain3/1
  Band-Limited White Noise/1 -> Gain/1
  Sum1/1 -> Zero-Order Hold/1
  Zero-Order Hold/1 -> u + n/1

== system AutomotiveEMS/v_l sensor/Voltage Sensor/Ideal voltage sensor ==
  PS-Simulink Converter : nesl_utility/PS-Simulink Converter  PhysicalDomain=network_engine_domain  SubClassName=ps_output  LeftPortType=input  RightPortType=output  PseudoPeriodic=off  Frequencies=[]  Unit=1  AffineConversion=off
  Voltage Sensor : fl_lib/Electrical/Electrical Sensors/Voltage Sensor
  + : PMIOPort  Side=Left
  - : PMIOPort  Port=2  Side=Right
  v : Outport
  wires:
  PS-Simulink Converter/1 -> v/1
  connections:
  Voltage Sensor/LConn1 -- +/RConn1
  -/RConn1 -- Voltage Sensor/RConn2
  Voltage Sensor/RConn1 -- PS-Simulink Converter/LConn1

== system AutomotiveEMS/v_l sensor/Voltage Sensor/Noise addition ==
  u : Inport
  Band-Limited White Noise : simulink/Sources/Band-Limited White Noise  Cov=[0.1]  Ts=T_s  seed=[seed]
  Gain : Gain  Gain=1/100
  Gain3 : Gain  Gain=noise
  Product2 : Product
  Sum1 : Sum  Inputs=|++
  Zero-Order Hold : ZeroOrderHold  SampleTime=T_s
  u + n : Outport
  wires:
  Gain3/1 -> Product2/1
  Product2/1 -> Sum1/1
  Gain/1 -> Product2/2
  u/1 -> Sum1/2, Gain3/1
  Band-Limited White Noise/1 -> Gain/1
  Sum1/1 -> Zero-Order Hold/1
  Zero-Order Hold/1 -> u + n/1

== system AutomotiveEMS/v_uc sensor/Voltage Sensor/Ideal voltage sensor ==
  PS-Simulink Converter : nesl_utility/PS-Simulink Converter  PhysicalDomain=network_engine_domain  SubClassName=ps_output  LeftPortType=input  RightPortType=output  PseudoPeriodic=off  Frequencies=[]  Unit=1  AffineConversion=off
  Voltage Sensor : fl_lib/Electrical/Electrical Sensors/Voltage Sensor
  + : PMIOPort  Side=Left
  - : PMIOPort  Port=2  Side=Right
  v : Outport
  wires:
  PS-Simulink Converter/1 -> v/1
  connections:
  Voltage Sensor/LConn1 -- +/RConn1
  -/RConn1 -- Voltage Sensor/RConn2
  Voltage Sensor/RConn1 -- PS-Simulink Converter/LConn1

== system AutomotiveEMS/v_uc sensor/Voltage Sensor/Noise addition ==
  u : Inport
  Band-Limited White Noise : simulink/Sources/Band-Limited White Noise  Cov=[0.1]  Ts=T_s  seed=[seed]
  Gain : Gain  Gain=1/100
  Gain3 : Gain  Gain=noise
  Product2 : Product
  Sum1 : Sum  Inputs=|++
  Zero-Order Hold : ZeroOrderHold  SampleTime=T_s
  u + n : Outport
  wires:
  Gain3/1 -> Product2/1
  Product2/1 -> Sum1/1
  Gain/1 -> Product2/2
  u/1 -> Sum1/2, Gain3/1
  Band-Limited White Noise/1 -> Gain/1
  Sum1/1 -> Zero-Order Hold/1
  Zero-Order Hold/1 -> u + n/1

== system AutomotiveEMS/Alternator/Armature circuit/Armature circuit (Delta)/i_a sensor ==
  Current Sensor : fl_lib/Electrical/Electrical Sensors/Current Sensor
  PS-Simulink Converter : nesl_utility/PS-Simulink Converter  PhysicalDomain=network_engine_domain  SubClassName=ps_output  LeftPortType=input  RightPortType=output  PseudoPeriodic=off  Frequencies=[]  Unit=1  AffineConversion=off
  + : PMIOPort  Side=Left
  - : PMIOPort  Port=2  Side=Right
  i : Outport
  wires:
  PS-Simulink Converter/1 -> i/1
  connections:
  Current Sensor/RConn2 -- -/RConn1
  Current Sensor/LConn1 -- +/RConn1
  PS-Simulink Converter/LConn1 -- Current Sensor/RConn1

== system AutomotiveEMS/Alternator/Armature circuit/Armature circuit (Delta)/i_b sensor ==
  Current Sensor : fl_lib/Electrical/Electrical Sensors/Current Sensor
  PS-Simulink Converter : nesl_utility/PS-Simulink Converter  PhysicalDomain=network_engine_domain  SubClassName=ps_output  LeftPortType=input  RightPortType=output  PseudoPeriodic=off  Frequencies=[]  Unit=1  AffineConversion=off
  + : PMIOPort  Side=Left
  - : PMIOPort  Port=2  Side=Right
  i : Outport
  wires:
  PS-Simulink Converter/1 -> i/1
  connections:
  Current Sensor/RConn2 -- -/RConn1
  Current Sensor/LConn1 -- +/RConn1
  PS-Simulink Converter/LConn1 -- Current Sensor/RConn1

== system AutomotiveEMS/Alternator/Armature circuit/Armature circuit (Delta)/i_c sensor ==
  Current Sensor : fl_lib/Electrical/Electrical Sensors/Current Sensor
  PS-Simulink Converter : nesl_utility/PS-Simulink Converter  PhysicalDomain=network_engine_domain  SubClassName=ps_output  LeftPortType=input  RightPortType=output  PseudoPeriodic=off  Frequencies=[]  Unit=1  AffineConversion=off
  + : PMIOPort  Side=Left
  - : PMIOPort  Port=2  Side=Right
  i : Outport
  wires:
  PS-Simulink Converter/1 -> i/1
  connections:
  Current Sensor/RConn2 -- -/RConn1
  Current Sensor/LConn1 -- +/RConn1
  PS-Simulink Converter/LConn1 -- Current Sensor/RConn1

== system AutomotiveEMS/Alternator/Armature circuit/Armature circuit (Delta)/r_a ==
  Constant : Constant  Value=r_ref
  Constant1 : Constant  Value=T_ref
  Constant2 : Constant  Value=T
  Constant3 : Constant  Value=alpha
  MATLAB Function : MATLAB Function  TreatAsAtomicUnit=on
  R : fl_lib/Electrical/Electrical Elements/Variable Resistor  Rmin=0 Ohm  i_specify=off  i_priority=None  i=0 A  i_nominal_specify=off  i_nominal_unit=A  i_nominal_value=1  v_specify=off  v_priority=None  v=0 V  v_nominal_specify=off  v_nominal_unit=V  v_nominal_value=1
  Simulink-PS Converter : nesl_utility/Simulink-PS Converter  PhysicalDomain=network_engine_domain  SubClassName=ps_input  LeftPortType=input  RightPortType=output  PseudoPeriodic=off  Frequencies=[]  NoiseDistribution=none  NoiseParameters=[]  Unit=1  AffineConversion=off  FilteringAndDerivatives=provide  SimscapeFilterOrder=1  InputFilterTimeConstant=0.001  UdotUserProvided=0
  + : PMIOPort  Side=Left
  - : PMIOPort  Port=2  Side=Right
  wires:
  MATLAB Function/1(r) -> Simulink-PS Converter/1
  Constant/1 -> MATLAB Function/1(r_ref)
  Constant1/1 -> MATLAB Function/2(T_ref)
  Constant3/1 -> MATLAB Function/4(alpha)
  Constant2/1 -> MATLAB Function/3(T)
  connections:
  Simulink-PS Converter/RConn1 -- R/LConn1
  R/RConn1 -- -/RConn1
  R/LConn2 -- +/RConn1

== system AutomotiveEMS/Alternator/Armature circuit/Armature circuit (Delta)/r_b ==
  Constant : Constant  Value=r_ref
  Constant1 : Constant  Value=T_ref
  Constant2 : Constant  Value=T
  Constant3 : Constant  Value=alpha
  MATLAB Function : MATLAB Function  TreatAsAtomicUnit=on
  R : fl_lib/Electrical/Electrical Elements/Variable Resistor  Rmin=0 Ohm  i_specify=off  i_priority=None  i=0 A  i_nominal_specify=off  i_nominal_unit=A  i_nominal_value=1  v_specify=off  v_priority=None  v=0 V  v_nominal_specify=off  v_nominal_unit=V  v_nominal_value=1
  Simulink-PS Converter : nesl_utility/Simulink-PS Converter  PhysicalDomain=network_engine_domain  SubClassName=ps_input  LeftPortType=input  RightPortType=output  PseudoPeriodic=off  Frequencies=[]  NoiseDistribution=none  NoiseParameters=[]  Unit=1  AffineConversion=off  FilteringAndDerivatives=provide  SimscapeFilterOrder=1  InputFilterTimeConstant=0.001  UdotUserProvided=0
  + : PMIOPort  Side=Left
  - : PMIOPort  Port=2  Side=Right
  wires:
  MATLAB Function/1(r) -> Simulink-PS Converter/1
  Constant/1 -> MATLAB Function/1(r_ref)
  Constant1/1 -> MATLAB Function/2(T_ref)
  Constant3/1 -> MATLAB Function/4(alpha)
  Constant2/1 -> MATLAB Function/3(T)
  connections:
  Simulink-PS Converter/RConn1 -- R/LConn1
  R/RConn1 -- -/RConn1
  R/LConn2 -- +/RConn1

== system AutomotiveEMS/Alternator/Armature circuit/Armature circuit (Delta)/r_c ==
  Constant : Constant  Value=r_ref
  Constant1 : Constant  Value=T_ref
  Constant2 : Constant  Value=T
  Constant3 : Constant  Value=alpha
  MATLAB Function : MATLAB Function  TreatAsAtomicUnit=on
  R : fl_lib/Electrical/Electrical Elements/Variable Resistor  Rmin=0 Ohm  i_specify=off  i_priority=None  i=0 A  i_nominal_specify=off  i_nominal_unit=A  i_nominal_value=1  v_specify=off  v_priority=None  v=0 V  v_nominal_specify=off  v_nominal_unit=V  v_nominal_value=1
  Simulink-PS Converter : nesl_utility/Simulink-PS Converter  PhysicalDomain=network_engine_domain  SubClassName=ps_input  LeftPortType=input  RightPortType=output  PseudoPeriodic=off  Frequencies=[]  NoiseDistribution=none  NoiseParameters=[]  Unit=1  AffineConversion=off  FilteringAndDerivatives=provide  SimscapeFilterOrder=1  InputFilterTimeConstant=0.001  UdotUserProvided=0
  + : PMIOPort  Side=Left
  - : PMIOPort  Port=2  Side=Right
  wires:
  MATLAB Function/1(r) -> Simulink-PS Converter/1
  Constant/1 -> MATLAB Function/1(r_ref)
  Constant1/1 -> MATLAB Function/2(T_ref)
  Constant3/1 -> MATLAB Function/4(alpha)
  Constant2/1 -> MATLAB Function/3(T)
  connections:
  Simulink-PS Converter/RConn1 -- R/LConn1
  R/RConn1 -- -/RConn1
  R/LConn2 -- +/RConn1

== system AutomotiveEMS/Alternator/Armature circuit/Armature circuit (Delta)/v_a sensor ==
  PS-Simulink Converter : nesl_utility/PS-Simulink Converter  PhysicalDomain=network_engine_domain  SubClassName=ps_output  LeftPortType=input  RightPortType=output  PseudoPeriodic=off  Frequencies=[]  Unit=1  AffineConversion=off
  Voltage Sensor : fl_lib/Electrical/Electrical Sensors/Voltage Sensor
  + : PMIOPort  Side=Left
  - : PMIOPort  Port=2  Side=Right
  v : Outport
  wires:
  PS-Simulink Converter/1 -> v/1
  connections:
  Voltage Sensor/LConn1 -- +/RConn1
  -/RConn1 -- Voltage Sensor/RConn2
  Voltage Sensor/RConn1 -- PS-Simulink Converter/LConn1

== system AutomotiveEMS/Alternator/Armature circuit/Armature circuit (Delta)/v_b sensor ==
  PS-Simulink Converter : nesl_utility/PS-Simulink Converter  PhysicalDomain=network_engine_domain  SubClassName=ps_output  LeftPortType=input  RightPortType=output  PseudoPeriodic=off  Frequencies=[]  Unit=1  AffineConversion=off
  Voltage Sensor : fl_lib/Electrical/Electrical Sensors/Voltage Sensor
  + : PMIOPort  Side=Left
  - : PMIOPort  Port=2  Side=Right
  v : Outport
  wires:
  PS-Simulink Converter/1 -> v/1
  connections:
  Voltage Sensor/LConn1 -- +/RConn1
  -/RConn1 -- Voltage Sensor/RConn2
  Voltage Sensor/RConn1 -- PS-Simulink Converter/LConn1

== system AutomotiveEMS/Alternator/Armature circuit/Armature circuit (Delta)/v_c sensor ==
  PS-Simulink Converter : nesl_utility/PS-Simulink Converter  PhysicalDomain=network_engine_domain  SubClassName=ps_output  LeftPortType=input  RightPortType=output  PseudoPeriodic=off  Frequencies=[]  Unit=1  AffineConversion=off
  Voltage Sensor : fl_lib/Electrical/Electrical Sensors/Voltage Sensor
  + : PMIOPort  Side=Left
  - : PMIOPort  Port=2  Side=Right
  v : Outport
  wires:
  PS-Simulink Converter/1 -> v/1
  connections:
  Voltage Sensor/LConn1 -- +/RConn1
  -/RConn1 -- Voltage Sensor/RConn2
  Voltage Sensor/RConn1 -- PS-Simulink Converter/LConn1

== system AutomotiveEMS/Alternator/Armature circuit/Armature circuit (Y)/i_a sensor ==
  Current Sensor : fl_lib/Electrical/Electrical Sensors/Current Sensor
  PS-Simulink Converter : nesl_utility/PS-Simulink Converter  PhysicalDomain=network_engine_domain  SubClassName=ps_output  LeftPortType=input  RightPortType=output  PseudoPeriodic=off  Frequencies=[]  Unit=1  AffineConversion=off
  + : PMIOPort  Side=Left
  - : PMIOPort  Port=2  Side=Right
  i : Outport
  wires:
  PS-Simulink Converter/1 -> i/1
  connections:
  Current Sensor/RConn2 -- -/RConn1
  Current Sensor/LConn1 -- +/RConn1
  PS-Simulink Converter/LConn1 -- Current Sensor/RConn1

== system AutomotiveEMS/Alternator/Armature circuit/Armature circuit (Y)/i_b sensor ==
  Current Sensor : fl_lib/Electrical/Electrical Sensors/Current Sensor
  PS-Simulink Converter : nesl_utility/PS-Simulink Converter  PhysicalDomain=network_engine_domain  SubClassName=ps_output  LeftPortType=input  RightPortType=output  PseudoPeriodic=off  Frequencies=[]  Unit=1  AffineConversion=off
  + : PMIOPort  Side=Left
  - : PMIOPort  Port=2  Side=Right
  i : Outport
  wires:
  PS-Simulink Converter/1 -> i/1
  connections:
  Current Sensor/RConn2 -- -/RConn1
  Current Sensor/LConn1 -- +/RConn1
  PS-Simulink Converter/LConn1 -- Current Sensor/RConn1

== system AutomotiveEMS/Alternator/Armature circuit/Armature circuit (Y)/i_c sensor ==
  Current Sensor : fl_lib/Electrical/Electrical Sensors/Current Sensor
  PS-Simulink Converter : nesl_utility/PS-Simulink Converter  PhysicalDomain=network_engine_domain  SubClassName=ps_output  LeftPortType=input  RightPortType=output  PseudoPeriodic=off  Frequencies=[]  Unit=1  AffineConversion=off
  + : PMIOPort  Side=Left
  - : PMIOPort  Port=2  Side=Right
  i : Outport
  wires:
  PS-Simulink Converter/1 -> i/1
  connections:
  Current Sensor/RConn2 -- -/RConn1
  Current Sensor/LConn1 -- +/RConn1
  PS-Simulink Converter/LConn1 -- Current Sensor/RConn1
